simulink model "torqueBalancingPHRIStandup"  (Simulink 9.1)
settings: Solver=FixedStepDiscrete  StartTime=0.0  StopTime="Config.SIMULATION_TIME "  FixedStep=Config.Ts  RelTol=1e-3  EnableMultiTasking=on
InitFcn:
  | cd(fileparts(which(bdroot)));
  | initTorqueBalancingPHRIStandup;
StopFcn:
  | cd(fileparts(which(bdroot)));
  | stopTorqueBalancingPHRIStandup;
undefined symbols (not defined in the file or in its folder): bVectorConstraintsFeet, bVectorConstraintsLegs, Config, ConstraintsMatrixFeet, ConstraintsMatrixLegs, Gain, HUMAN_DOF_FOR_SIMULINK, Reg, ROBOT_DOF, ROBOT_DOF_FOR_SIMULINK, Sat, Sm
libraries: WBToolboxLibrary x153, simulink x4
(part 4 of 4)

== matlab function Robot system/controller_QP/Balancing Controller  ==
  data: tauModel output double; Sigma output double; NA output double; f_HDot output double; HessianMatrixQP1Foot output double; gradientQP1Foot output double; ConstraintsMatrixQP1Foot output double; bVectorConstraintsQp1Foot output double; HessianMatrixQP2FeetOrLegs output double; gradientQP2FeetOrLegs output double; ConstraintsMatrixQP2FeetOrLegs output double; bVectorConstraintsQp2FeetOrLegs output double; constraints input double; ROBOT_DOF_FOR_SIMULINK input double; HUMAN_DOF_FOR_SIMULINK input double; ConstraintsMatrix input double; bVectorConstraints input double; qj input double; qjDes input double; nu input double; M input double; h input double; L input double; intLw input double; w_H_l_contact input double; w_H_r_contact input double; JL input double; JR input double; dJL_nu input double; dJR_nu input double; xCoM input double; J_CoM input double; desired_x_dx_ddx_CoM input double; CMM input double; gainsPCOM input double; gainsDCOM input double; impedances input double; Reg parameter double; errorCoM output double; f_noQP output double; Gain parameter double; w_H_lArm input double; w_H_rArm input double; JLArm input double; JRArm input double; dJLArm_nu input double; dJRArm_nu input double; LArmWrench input double; RArmWrench input double; STANDUP_WITH_HUMAN_FORCE input double; MEASURED_FT input double; STANDUP_WITH_HUMAN_TORQUE input double; human_w_H_b input double; human_qj input double; human_nu_b input double; human_dqj input double; human_M input double; human_h input double; human_torques input double; human_w_H_l_contact input double; human_w_H_r_contact input double; human_JL input double; human_JR input double; human_dJL_nu input double; human_dJR_nu input double; human_w_H_lArm_contact input double; human_w_H_rArm_contact input double; human_JLArm input double; human_JRArm input double; human_dJLArm_nu input double; human_dJRArm_nu input double; correctionFromSupportForce output double; L_error output double; V output double; alpha output double; state input double; robot_torques input double; fArms output double; phri_human_feet_wrench output double; phri_robot_feet_wrench output double; correctionFromSupportTorque output double
function [tauModel, Sigma, NA, f_HDot, ...
          HessianMatrixQP1Foot, gradientQP1Foot, ConstraintsMatrixQP1Foot, bVectorConstraintsQp1Foot, ...
          HessianMatrixQP2FeetOrLegs, gradientQP2FeetOrLegs, ConstraintsMatrixQP2FeetOrLegs, bVectorConstraintsQp2FeetOrLegs, ...
          errorCoM, f_noQP, correctionFromSupportForce, L_error, V, alpha, fArms, phri_human_feet_wrench, phri_robot_feet_wrench, correctionFromSupportTorque] =  ...
              balancingControllerStandupFCN(constraints, ROBOT_DOF_FOR_SIMULINK, HUMAN_DOF_FOR_SIMULINK, ConstraintsMatrix, bVectorConstraints, ...
                                         qj, qjDes, nu, M, h, L, intLw, w_H_l_contact, w_H_r_contact, JL, JR, dJL_nu, dJR_nu, xCoM, J_CoM, desired_x_dx_ddx_CoM, CMM, ...
                                         gainsPCOM, gainsDCOM, impedances, Reg, Gain, w_H_lArm, w_H_rArm, JLArm, JRArm, dJLArm_nu, dJRArm_nu,...
                                         LArmWrench, RArmWrench, STANDUP_WITH_HUMAN_FORCE, MEASURED_FT, STANDUP_WITH_HUMAN_TORQUE, ...
                                         human_w_H_b, human_qj, human_nu_b, human_dqj, human_M, human_h, human_torques, ...
                                         human_w_H_l_contact, human_w_H_r_contact, human_JL, human_JR, human_dJL_nu, human_dJR_nu,...
                                         human_w_H_lArm_contact, human_w_H_rArm_contact, human_JLArm, human_JRArm, human_dJLArm_nu, human_dJRArm_nu,...
                                         state, robot_torques)
           
   [tauModel, Sigma, NA, f_HDot, ...
          HessianMatrixQP1Foot, gradientQP1Foot, ConstraintsMatrixQP1Foot, bVectorConstraintsQp1Foot, ...
          HessianMatrixQP2FeetOrLegs, gradientQP2FeetOrLegs, ConstraintsMatrixQP2FeetOrLegs, bVectorConstraintsQp2FeetOrLegs, ...
          errorCoM, f_noQP, correctionFromSupportForce, L_error, V, alpha, fArms, phri_human_feet_wrench, phri_robot_feet_wrench, correctionFromSupportTorque] =  ...
              balancingControllerStandup(constraints, ROBOT_DOF_FOR_SIMULINK, HUMAN_DOF_FOR_SIMULINK, ConstraintsMatrix, bVectorConstraints, ...
                                         qj, qjDes, nu, M, h, L, intLw, w_H_l_contact, w_H_r_contact, JL, JR, dJL_nu, dJR_nu, xCoM, J_CoM, desired_x_dx_ddx_CoM, CMM, ...
                                         gainsPCOM, gainsDCOM, impedances, Reg, Gain, w_H_lArm, w_H_rArm, JLArm, JRArm, dJLArm_nu, dJRArm_nu,...
                                         LArmWrench, RArmWrench, STANDUP_WITH_HUMAN_FORCE, MEASURED_FT, STANDUP_WITH_HUMAN_TORQUE, ...
                                         human_w_H_b, human_qj, human_nu_b, human_dqj, human_M, human_h, human_torques, ...
                                         human_w_H_l_contact, human_w_H_r_contact, human_JL, human_JR, human_dJL_nu, human_dJR_nu,...
                                         human_w_H_lArm_contact, human_w_H_rArm_contact, human_JLArm, human_JRArm, human_dJLArm_nu, human_dJRArm_nu,...
                                         state, robot_torques);
end

== matlab function Robot system/emergency stop: joint limits/MATLAB Function ==
  data: umin input double; umax input double; u input double; inRange output double; tol input double
function inRange = checkRangeFCN(umin, umax, u, tol)

    inRange = checkRange(umin, umax, u, tol);
end

== matlab function Robot system/controller_QP/Compute angular momentum integral/References for H ==
  data: qjErr input double; JL input double; JR input double; nu_b_equivalent output double; Reg parameter double; activeFeetConstraints input double
function nu_b_equivalent = generateReferencesForH_FCN(qjErr, JL, JR, Reg, activeFeetConstraints)

    if activeFeetConstraints(1) == 1
    
        pinvJb          = (JL(:,1:6)'*JL(:,1:6) + Reg.pinvDamp_nu_b*eye(6))\JL(:,1:6)';
        nu_b_equivalent = -pinvJb*JL(:,7:end)*qjErr;
    else
    
        pinvJb          = (JR(:,1:6)'*JR(:,1:6) + Reg.pinvDamp_nu_b*eye(6))\JR(:,1:6)';
        nu_b_equivalent = -pinvJb*JR(:,7:end)*qjErr;
    end
end

== matlab function Robot system/Robot State and References/State Machine Standup/Visualise extrnal wrenches/Compute current threshold ==
  data: thresholdContactLeftHand output double; thresholdContactRightHand output double; state input double; thresholdContactLeftFoot output double; thresholdContactRightFoot output double; Sm parameter double
function [thresholdContactLeftHand,thresholdContactRightHand, ...
          thresholdContactLeftFoot,thresholdContactRightFoot] = currentThreshold(state,Sm)

    thresholdContactLeftHand  = Sm.wrench_thresholdContactLHand(state);
    thresholdContactRightHand = Sm.wrench_thresholdContactRHand(state);
    thresholdContactLeftFoot  = Sm.wrench_thresholdContactLFoot(state);
    thresholdContactRightFoot = Sm.wrench_thresholdContactRFoot(state);
end
